simulink library "app"  (R2021b)
settings: Solver=VariableStepAuto  StartTime=0.0  StopTime=10.0  RelTol=1e-3
undefined symbols (not defined in the file): C_TASK_10MS_S, C_TASK_5MS_S, slcm
libraries: acc x1, apm x1, bcm x1, ddm x1, dhp x1, dkc x1, dsc x1, nmm x1, pmm x1, scp x1, sys x1, thc x1
settings Model: Creator=jc19  LastModifiedBy=FVT22115
settings SolverCC: AlgebraicLoopSolver=TrustRegion
settings DataIOCC: SaveFormat=Array  SignalLoggingSaveFormat=ModelDataLogs  ReturnWorkspaceOutputs=off
settings OptimizationCC: BlockReduction=off  BooleanDataType=off
settings DebuggingCC: SaveWithParameterizedLinksMsg=none  UnderspecifiedInitializationDetection=Classic  MergeDetectMultiDrivingBlocksExec=none  SignalResolutionControl=TryResolveAllWithWarning  SFMachineParentedDataDiag=warning
settings HardwareCC: TargetUnknown=on
settings ModelReferenceCC: PropagateSignalLabelsOutOfModel=off
settings SFSimCC: SimUseLocalCustomCode=off
settings RTWCC: RTWUseLocalCustomCode=off
settings ConfigComp: CovMetricSettings=dw  CovSaveCumulativeToWorkspaceVar=on  CovSaveSingleToWorkspaceVar=on

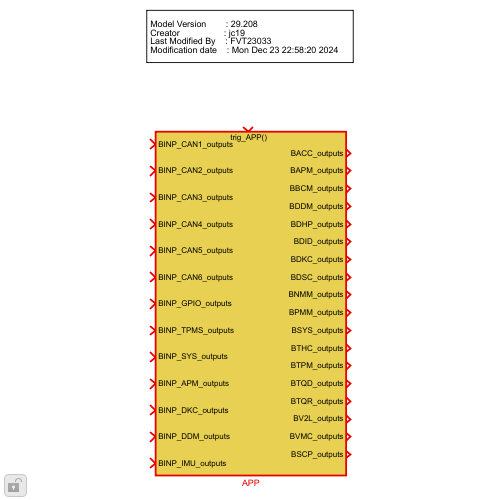
[thumbnail: Simulink's stored preview of the top-level diagram]
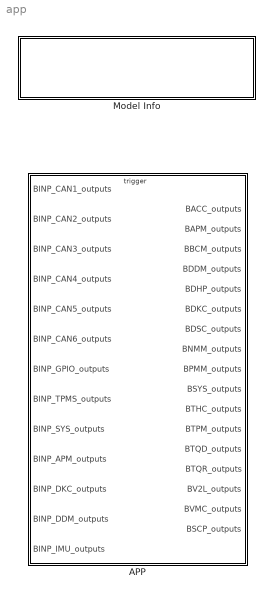
== system app ==
  APP : Subsystem
  Model Info : Subsystem  LoadFcn=slcm LoadBlock;  InitFcn=slcm('UpdateAllCMBlocksInThisModelInit')  mask(CMBlock){InitialSaveTempField=, InitialBlockCM=None, BlockCM=None, Frame=on, SaveTempField=, DisplayStringWithTags=|, MaskDisplayString=Model Version        : 29.221\nCreator                  : jc19\nLast Modified By    : FVT23131\nModification date    : Fri Apr 18 09:47:03 2025, HorizontalTextAlignment=Left, LeftAlignmentValue=0.02, SourceBlockDiagram=app, TagMaxNumber=20, CMTag1=, CMTag2=, CMTag3=, CMTag4=, CMTag5=, CMTag6=, CMTag7=, CMTag8=, CMTag9=, CMTag10=, CMTag11=, CMTag12=, CMTag13=, CMTag14=, CMTag15=, CMTag16=, CMTag17=, CMTag18=, CMTag19=, CMTag20=}
      mask DisplayStringWithTags=|
      | Model Version        : %<ModelVersion>
      | Creator                  : %<Creator>
      | Last Modified By    : %<LastModifiedBy>
      | Modification date    : %<LastModificationDate>
      mask help: This block allows revision control information to be displayed within the model.
      settings: CopyFcn=slcm CopyBlock;  DeleteFcn=slcm Cancel;  PostSaveFcn=slcm('UpdateAllCMBlocksInThisModel')  NameChangeFcn=slcm Rename;  OpenFcn=slcm
      mask Display: text(str2num(LeftAlignmentValue), 0.5, MaskDisplayString, 'HorizontalAlignment', HorizontalTextAlignment)

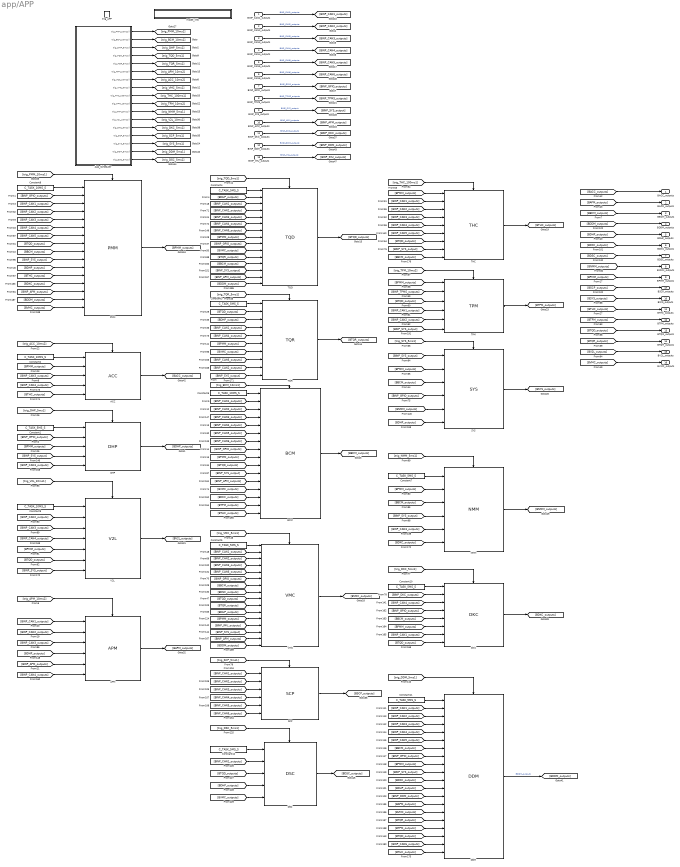
== system app/APP ==
  BINP_CAN1_outputs : Inport  OutDataTypeStr=Bus: BINP_CAN1_outputs
  BINP_CAN2_outputs : Inport  Port=2  OutDataTypeStr=Bus: BINP_CAN2_outputs
  BINP_CAN3_outputs : Inport  Port=3  OutDataTypeStr=Bus: BINP_CAN3_outputs
  BINP_CAN4_outputs : Inport  Port=4  OutDataTypeStr=Bus: BINP_CAN4_outputs
  BINP_CAN5_outputs : Inport  Port=5  OutDataTypeStr=Bus: BINP_CAN5_outputs
  BINP_CAN6_outputs : Inport  Port=6  OutDataTypeStr=Bus: BINP_CAN6_outputs
  BINP_GPIO_outputs : Inport  Port=7  OutDataTypeStr=Bus: BINP_GPIO_outputs
  BINP_TPMS_outputs : Inport  Port=8  OutDataTypeStr=Bus: BINP_TPMS_outputs
  BINP_SYS_outputs : Inport  Port=9  OutDataTypeStr=Bus: BINP_SYS_outputs
  BINP_APM_outputs : Inport  Port=10  OutDataTypeStr=Bus: BINP_APM_outputs
  BINP_DKC_outputs : Inport  Port=11  OutDataTypeStr=Bus: BINP_DKC_outputs
  BINP_DDM_outputs : Inport  Port=12  OutDataTypeStr=Bus: BINP_DDM_outputs
  BINP_IMU_outputs : Inport  Port=13  OutDataTypeStr=Bus: BINP_IMU_outputs
  trig_APP : TriggerPort  TriggerType=function-call  VariantControl=(inherit)
  ACC : acc/ACC  SystemSampleTime=-1  VariantActivationTime=update diagram  Latency=0  AutoFrameSizeCalculation=off
  APM : apm/APM  SystemSampleTime=-1  VariantActivationTime=update diagram  Latency=0  AutoFrameSizeCalculation=off
  App_Scheduler : Stateflow chart  TreatAsAtomicUnit=on
  BCM : bcm/BCM  SystemSampleTime=-1  VariantActivationTime=update diagram  Latency=0  AutoFrameSizeCalculation=off
  Constant{1,3..5,7,10..12} (8 alike) : Constant  Value=C_TASK_5MS_S  OutDataTypeStr=single
  Constant{2,6,8..9} (4 alike) : Constant  Value=C_TASK_10MS_S  OutDataTypeStr=single
  DDM : ddm/DDM  SystemSampleTime=-1  VariantActivationTime=update diagram  Latency=0  AutoFrameSizeCalculation=off
  DHP : dhp/DHP  SystemSampleTime=-1  VariantActivationTime=update diagram  Latency=0  AutoFrameSizeCalculation=off
  DKC : dkc/DKC  SystemSampleTime=-1  VariantActivationTime=update diagram  Latency=0  AutoFrameSizeCalculation=off
  DSC : dsc/DSC  SystemSampleTime=-1  VariantActivationTime=update diagram  Latency=0  AutoFrameSizeCalculation=off
  NMM : nmm/NMM  SystemSampleTime=-1  VariantActivationTime=update diagram  Latency=0  AutoFrameSizeCalculation=off
  PMM : pmm/PMM  SystemSampleTime=-1  VariantActivationTime=update diagram  Latency=0  AutoFrameSizeCalculation=off
  SCP : scp/SCP  SystemSampleTime=-1  VariantActivationTime=update diagram  Latency=0  AutoFrameSizeCalculation=off
  SYS : sys/SYS  SystemSampleTime=-1  VariantActivationTime=update diagram  Latency=0  AutoFrameSizeCalculation=off
  THC : thc/THC  SystemSampleTime=-1  VariantActivationTime=update diagram  Latency=0  AutoFrameSizeCalculation=off
  TPM : tpm/TPM  SystemSampleTime=-1  VariantActivationTime=update diagram  Latency=0  AutoFrameSizeCalculation=off
  TQD : tqd/TQD  SystemSampleTime=-1  VariantActivationTime=update diagram  Latency=0  AutoFrameSizeCalculation=off
  TQR : tqr/TQR  SystemSampleTime=-1  VariantActivationTime=update diagram  Latency=0  AutoFrameSizeCalculation=off
  V2L : v2l/V2L  SystemSampleTime=-1  VariantActivationTime=update diagram  Latency=0  AutoFrameSizeCalculation=off
  VMC : vmc/VMC  SystemSampleTime=-1  VariantActivationTime=update diagram  Latency=0  AutoFrameSizeCalculation=off
  model_info : Subsystem  LoadFcn=slcm LoadBlock;  InitFcn=slcm('UpdateAllCMBlocksInThisModelInit')  mask(CMBlock){InitialSaveTempField=, InitialBlockCM=None, BlockCM=None, Frame=on, SaveTempField=, DisplayStringWithTags=$Id: app.mdl 2023 2013-03-20 03:40:02Z wxia $, MaskDisplayString=$Id: app.mdl 2023 2013-03-20 03:40:02Z wxia $, HorizontalTextAlignment=Center, LeftAlignmentValue=0.5, SourceBlockDiagram=app, TagMaxNumber=20, CMTag1=, CMTag2=, CMTag3=, CMTag4=, CMTag5=, CMTag6=, CMTag7=, CMTag8=, CMTag9=, CMTag10=, CMTag11=, CMTag12=, CMTag13=, CMTag14=, CMTag15=, CMTag16=, CMTag17=, CMTag18=, CMTag19=, CMTag20=}
      mask help: This block allows revision control information to be displayed within the model.
      settings: CopyFcn=slcm CopyBlock;  DeleteFcn=slcm Cancel;  PostSaveFcn=slcm('UpdateAllCMBlocksInThisModel')  NameChangeFcn=slcm Rename;  OpenFcn=slcm
      mask Display: text(str2num(LeftAlignmentValue), 0.5, MaskDisplayString, 'HorizontalAlignment', HorizontalTextAlignment)
  BACC_outputs : Outport  OutDataTypeStr=Bus: BACC_outputs  VectorParamsAs1DForOutWhenUnconnected=off
  BAPM_outputs : Outport  Port=2  OutDataTypeStr=Bus: BAPM_outputs
  BBCM_outputs : Outport  Port=3  OutDataTypeStr=Bus: BBCM_outputs  VectorParamsAs1DForOutWhenUnconnected=off
  BDDM_outputs : Outport  Port=4  OutDataTypeStr=Bus: BDDM_outputs  VectorParamsAs1DForOutWhenUnconnected=off
  BDHP_outputs : Outport  Port=5  OutDataTypeStr=Bus: BDHP_outputs  VectorParamsAs1DForOutWhenUnconnected=off
  BDKC_outputs : Outport  Port=6  OutDataTypeStr=Bus: BDKC_outputs  VectorParamsAs1DForOutWhenUnconnected=off
  BDSC_outputs : Outport  Port=7  OutDataTypeStr=Bus: BDSC_outputs  VectorParamsAs1DForOutWhenUnconnected=off
  BNMM_outputs : Outport  Port=8  OutDataTypeStr=Bus: BNMM_outputs  VectorParamsAs1DForOutWhenUnconnected=off
  BPMM_outputs : Outport  Port=9  OutDataTypeStr=Bus: BPMM_outputs  VectorParamsAs1DForOutWhenUnconnected=off
  BSYS_outputs : Outport  Port=10  OutDataTypeStr=Bus: BSYS_outputs  VectorParamsAs1DForOutWhenUnconnected=off
  BTHC_outputs : Outport  Port=11  OutDataTypeStr=Bus: BTHC_outputs  VectorParamsAs1DForOutWhenUnconnected=off
  BTPM_outputs : Outport  Port=12  OutDataTypeStr=Bus: BTPM_outputs  VectorParamsAs1DForOutWhenUnconnected=off
  BTQD_outputs : Outport  Port=13  OutDataTypeStr=Bus: BTQD_outputs  VectorParamsAs1DForOutWhenUnconnected=off
  BTQR_outputs : Outport  Port=14  OutDataTypeStr=Bus: BTQR_outputs  VectorParamsAs1DForOutWhenUnconnected=off
  BV2L_outputs : Outport  Port=15  OutDataTypeStr=Bus: BV2L_outputs  VectorParamsAs1DForOutWhenUnconnected=off
  BVMC_outputs : Outport  Port=16  OutDataTypeStr=Bus: BVMC_outputs  VectorParamsAs1DForOutWhenUnconnected=off
  BSCP_outputs : Outport  Port=17  OutDataTypeStr=Bus: BSCP_outputs  VectorParamsAs1DForOutWhenUnconnected=off
  wires:
  NMM/1 -> [BNMM_outputs]
  [trig_NMM_5ms1] -> NMM/Trigger
  Constant7/1 -> NMM/1
  DHP/1 -> [BDHP_outputs]
  Constant1/1 -> DHP/1
  [BINP_GPIO_outputs] -> DHP/2
  BINP_CAN1_outputs/1 -> [BINP_CAN1_outputs]  "BINP_CAN1_outputs"
  PMM/1 -> [BPMM_outputs]
  ACC/1 -> [BACC_outputs]
  [trig_PMM_10ms1] -> PMM/Trigger
  TQD/1 -> [BTQD_outputs]
  TQR/1 -> [BTQR_outputs]
  [BTQD_outputs] -> TQR/2
  Constant2/1 -> ACC/1
  [trig_BCM_10ms1] -> BCM/Trigger
  BCM/1 -> [BBCM_outputs]
  BINP_CAN2_outputs/1 -> [BINP_CAN2_outputs]  "BINP_CAN2_outputs"
  BINP_CAN3_outputs/1 -> [BINP_CAN3_outputs]  "BINP_CAN3_outputs"
  BINP_CAN4_outputs/1 -> [BINP_CAN4_outputs]  "BINP_CAN4_outputs"
  BINP_GPIO_outputs/1 -> [BINP_GPIO_outputs]  "BINP_GPIO_outputs"
  [trig_TQD_5ms1] -> TQD/Trigger
  [BPMM_outputs] -> DHP/3
  [trig_DHP_5ms1] -> DHP/Trigger
  BINP_CAN5_outputs/1 -> [BINP_CAN5_outputs]  "BINP_CAN5_outputs"
  [trig_TQR_5ms1] -> TQR/Trigger
  Constant3/1 -> TQR/1
  [BDHP_outputs] -> TQR/3
  [BINP_CAN1_outputs] -> TQR/4
  [trig_ACC_10ms2] -> ACC/Trigger
  [BINP_CAN3_outputs] -> ACC/3
  [BPMM_outputs] -> ACC/2
  [trig_VMC_5ms1] -> VMC/Trigger
  Constant5/1 -> VMC/1
  VMC/1 -> [BVMC_outputs]
  THC/1 -> [BTHC_outputs]
  [BPMM_outputs] -> THC/1
  [trig_THC_100ms1] -> THC/Trigger
  BINP_TPMS_outputs/1 -> [BINP_TPMS_outputs]  "BINP_TPMS_outputs"
  [trig_TPM_10ms2] -> TPM/Trigger
  [BPMM_outputs] -> TPM/1
  [BINP_TPMS_outputs] -> TPM/2
  [BTQD_outputs] -> TPM/3
  [BINP_CAN1_outputs] -> TPM/4
  [BINP_CAN2_outputs] -> TPM/5
  TPM/1 -> [BTPM_outputs]
  SYS/1 -> [BSYS_outputs]
  [BINP_CAN4_outputs] -> TQR/5
  [BPMM_outputs] -> TQR/6
  BINP_SYS_outputs/1 -> [BINP_SYS_output]  "BINP_SYS_output"
  Constant9/1 -> V2L/1
  [BINP_CAN3_outputs] -> V2L/3
  [BINP_CAN2_outputs] -> V2L/2
  [trig_V2L_10ms1] -> V2L/Trigger
  V2L/1 -> [BV2L_outputs]
  APM/1 -> [BAPM_outputs]
  [trig_APM_10ms2] -> APM/Trigger
  [BINP_CAN1_outputs] -> APM/1
  [BINP_CAN2_outputs] -> APM/2
  BINP_APM_outputs/1 -> [BINP_APM_outputs]  "BINP_APM_outputs"
  [trig_SYS_5ms1] -> SYS/Trigger
  [BINP_CAN3_outputs] -> APM/3
  [BVMC_outputs] -> TQR/7
  Constant8/1 -> PMM/1
  [BINP_CAN1_outputs] -> PMM/3
  [BINP_CAN4_outputs] -> PMM/6
  [BINP_GPIO_outputs] -> PMM/2
  [BINP_CAN3_outputs] -> PMM/5
  [BINP_CAN5_outputs] -> PMM/7
  [BTQD_outputs] -> PMM/8
  [BBCM_outputs] -> PMM/9
  [BINP_SYS_output] -> PMM/10
  [BINP_CAN2_outputs] -> PMM/4
  [BDHP_outputs] -> PMM/11
  [BPMM_outputs] -> NMM/2
  [BBCM_outputs] -> NMM/3
  [BINP_SYS_output] -> NMM/4
  [BTHC_outputs] -> PMM/12
  App_Scheduler/3(trig_DHP_5ms1()) -> [trig_DHP_5ms1]
  App_Scheduler/4(trig_TQD_5ms1()) -> [trig_TQD_5ms1]
  App_Scheduler/8(trig_VMC_5ms1()) -> [trig_VMC_5ms1]
  App_Scheduler/15(trig_SYS_5ms1()) -> [trig_SYS_5ms1]
  App_Scheduler/2(trig_BCM_10ms1()) -> [trig_BCM_10ms1]
  App_Scheduler/12(trig_V2L_10ms1()) -> [trig_V2L_10ms1]
  App_Scheduler/5(trig_TQR_5ms1()) -> [trig_TQR_5ms1]
  App_Scheduler/9(trig_THC_100ms1()) -> [trig_THC_100ms1]
  App_Scheduler/6(trig_APM_10ms2()) -> [trig_APM_10ms2]
  App_Scheduler/7(trig_ACC_10ms2()) -> [trig_ACC_10ms2]
  App_Scheduler/11(trig_NMM_5ms1()) -> [trig_NMM_5ms1]
  App_Scheduler/10(trig_TPM_10ms2()) -> [trig_TPM_10ms2]
  App_Scheduler/1(trig_PMM_10ms1()) -> [trig_PMM_10ms1]
  App_Scheduler/13(trig_DKC_5ms1()) -> [trig_DKC_5ms1]
  App_Scheduler/14(trig_SCP_5ms1()) -> [trig_SCP_5ms1]
  BINP_DKC_outputs/1 -> [BINP_DKC_outputs]  "BINP_DKC_outputs"
  [trig_DKC_5ms1] -> DKC/Trigger
  Constant10/1 -> DKC/1
  [BINP_DKC_outputs] -> DKC/2
  [BINP_CAN3_outputs] -> SCP/3
  [BINP_CAN2_outputs] -> SCP/2
  [BINP_CAN1_outputs] -> SCP/1
  [BINP_CAN4_outputs] -> SCP/4
  [BINP_CAN5_outputs] -> SCP/5
  [trig_SCP_5ms1] -> SCP/Trigger
  SCP/1 -> [BSCP_outputs]
  DKC/1 -> [BDKC_outputs]
  [BSYS_outputs] -> BSYS_outputs/1
  [BTQR_outputs] -> BTQR_outputs/1
  [BAPM_outputs] -> BAPM_outputs/1
  [BPMM_outputs] -> BPMM_outputs/1
  [BV2L_outputs] -> BV2L_outputs/1
  [BTQD_outputs] -> BTQD_outputs/1
  [BDHP_outputs] -> BDHP_outputs/1
  [BTPM_outputs] -> BTPM_outputs/1
  [BDKC_outputs] -> BDKC_outputs/1
  [BACC_outputs] -> BACC_outputs/1
  [BNMM_outputs] -> BNMM_outputs/1
  [BVMC_outputs] -> BVMC_outputs/1
  [BSCP_outputs] -> BSCP_outputs/1
  [BBCM_outputs] -> BBCM_outputs/1
  [BTHC_outputs] -> BTHC_outputs/1
  [BINP_SYS_output] -> SYS/1
  [BPMM_outputs] -> SYS/2
  [BBCM_outputs] -> SYS/3
  [BINP_GPIO_outputs] -> SYS/4
  App_Scheduler/16(trig_DDM_5ms1()) -> [trig_DDM_5ms1]
  [trig_DDM_5ms1] -> DDM/Trigger
  [BDDM_outputs] -> BDDM_outputs/1
  BINP_DDM_outputs/1 -> [BINP_DDM_outputs]  "BINP_DDM_outputs"
  [BINP_CAN1_outputs] -> VMC/2
  [BINP_CAN2_outputs] -> VMC/3
  [BINP_CAN3_outputs] -> VMC/4
  App_Scheduler/17(trig_DSC_5ms1()) -> [trig_DSC_5ms1]
  [trig_DSC_5ms1] -> DSC/Trigger
  Constant12/1 -> DSC/1
  [BINP_CAN1_outputs] -> DSC/2
  [BTQD_outputs] -> DSC/3
  [BDHP_outputs] -> DSC/4
  [BVMC_outputs] -> DSC/5
  DSC/1 -> [BDSC_outputs]
  BINP_CAN6_outputs/1 -> [BINP_CAN6_outputs]  "BINP_CAN6_outputs"
  [BDSC_outputs] -> BDSC_outputs/1
  Constant6/1 -> BCM/1
  [BINP_CAN1_outputs] -> BCM/2
  [BINP_CAN2_outputs] -> BCM/3
  Constant11/1 -> DDM/1
  [BINP_CAN1_outputs] -> DDM/2
  [BINP_CAN2_outputs] -> DDM/3
  [BINP_CAN3_outputs] -> DDM/4
  [BINP_CAN4_outputs] -> DDM/5
  [BINP_CAN5_outputs] -> DDM/6
  [BBCM_outputs] -> DDM/7
  [BINP_GPIO_outputs] -> DDM/8
  [BPMM_outputs] -> DDM/9
  [BINP_SYS_output] -> DDM/10
  [BDKC_outputs] -> DDM/11
  [BDHP_outputs] -> DDM/12
  [BINP_DDM_outputs] -> DDM/13
  [BAPM_outputs] -> DDM/14
  [BVMC_outputs] -> DDM/15
  [BTQR_outputs] -> DDM/16
  [BTPM_outputs] -> DDM/17
  [BINP_CAN3_outputs] -> NMM/5
  [BINP_CAN1_outputs] -> THC/2
  [BINP_CAN2_outputs] -> THC/3
  [BINP_CAN3_outputs] -> THC/4
  [BINP_CAN4_outputs] -> THC/5
  [BINP_SYS_output] -> THC/8
  [BTQD_outputs] -> THC/7
  [BINP_CAN5_outputs] -> THC/6
  [BINP_CAN4_outputs] -> DKC/3
  DDM/1 -> [BDDM_outputs]  "BDDM_outputs"
  BINP_IMU_outputs/1 -> [BINP_IMU_outputs]  "BINP_IMU_outputs"
  [BTQD_outputs] -> DDM/18
  [BNMM_outputs] -> SYS/5
  [BINP_CAN6_outputs] -> SCP/6
  [BINP_SYS_output] -> DHP/4
  Constant4/1 -> TQD/1
  [BDHP_outputs] -> TQD/2
  [BINP_CAN1_outputs] -> TQD/3
  [BINP_CAN2_outputs] -> TQD/4
  [BINP_CAN3_outputs] -> TQD/5
  [BINP_CAN4_outputs] -> TQD/6
  [BINP_CAN3_outputs] -> BCM/4
  [BINP_CAN4_outputs] -> BCM/5
  [BINP_CAN5_outputs] -> BCM/6
  [BINP_CAN6_outputs] -> BCM/7
  [BINP_GPIO_outputs] -> BCM/8
  [BPMM_outputs] -> BCM/9
  [BTQD_outputs] -> BCM/10
  [BINP_SYS_output] -> BCM/11
  [BINP_APM_outputs] -> BCM/12
  [BINP_APM_outputs] -> APM/5
  [BDHP_outputs] -> APM/4
  [BINP_CAN6_outputs] -> TQD/7
  [BPMM_outputs] -> TQD/8
  [BTQR_outputs] -> TQD/11
  [BINP_GPIO_outputs] -> TQD/9
  [BVMC_outputs] -> TQD/10
  [BBCM_outputs] -> TQD/12
  [BINP_SYS_output] -> TQD/13
  [BINP_CAN6_outputs] -> VMC/5
  [BINP_GPIO_outputs] -> VMC/6
  [BBCM_outputs] -> VMC/7
  [BDSC_outputs] -> VMC/8
  [BTQD_outputs] -> VMC/9
  [BTQR_outputs] -> VMC/10
  [BDHP_outputs] -> VMC/11
  [BPMM_outputs] -> VMC/12
  [BINP_IMU_outputs] -> VMC/13
  [BINP_SYS_output] -> VMC/14
  [BVMC_outputs] -> BCM/13
  [BDKC_outputs] -> BCM/14
  [BDKC_outputs] -> PMM/13
  [BTPM_outputs] -> BCM/15
  [BTHC_outputs] -> BCM/16
  [BINP_CAN6_outputs] -> TQR/8
  [BINP_APM_outputs] -> TQD/14
  [BINP_CAN3_outputs] -> DHP/5
  [BINP_CAN4_outputs] -> APM/6
  [BINP_APM_outputs] -> PMM/14
  [BINP_GPIO_outputs] -> DKC/4
  [BBCM_outputs] -> DKC/5
  [BPMM_outputs] -> DKC/6
  [BINP_CAN1_outputs] -> DKC/7
  [BTQD_outputs] -> DKC/8
  [BINP_APM_outputs] -> VMC/15
  [BINP_CAN2_outputs] -> TQR/9
  [BTQD_outputs] -> V2L/6
  [BPMM_outputs] -> V2L/5
  [BINP_CAN4_outputs] -> V2L/4
  [BINP_SYS_output] -> V2L/7
  [BDHP_outputs] -> SYS/6
  [BINP_SYS_output] -> TQR/10
  [BDKC_outputs] -> NMM/6
  [BDDM_outputs] -> TQD/15
  [BDDM_outputs] -> PMM/15
  [BVMC_outputs] -> PMM/16
  [BINP_CAN6_outputs] -> DDM/19
  [BDDM_outputs] -> VMC/16
  [BINP_SYS_output] -> TPM/6
  [BINP_CAN4_outputs] -> ACC/4
  [BTHC_outputs] -> ACC/5
  [BTHC_outputs] -> DDM/20
  [BBCM_outputs] -> THC/9

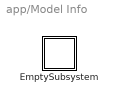
== system app/Model Info ==
  EmptySubsystem : Subsystem

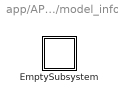
== system app/APP/model_info ==
  EmptySubsystem : Subsystem

== system app/Model Info/EmptySubsystem ==

== system app/APP/model_info/EmptySubsystem ==

== stateflow chart app/APP/App_Scheduler ==
  state Task_5_10_100ms
    (default) -> (junction 6) : {
        | counter = 0;
        | }
    Task_5_10_100ms -> (junction 6) : {
        | counter++;
        | }
    (junction 6) -> (junction 38) [order 1] : [counter%%2 == 0]  /* 10ms trigger #1*/
    (junction 6) -> (junction 44) [order 2]
    (junction 38) -> (junction 40) : {
        | trig_PMM_10ms1;
        | trig_BCM_10ms1;
        | trig_V2L_10ms1;
        | }
    (junction 40) -> (junction 44)
    (junction 44) -> (junction 63)
    (junction 63) -> (junction 107) [order 1] : %[VPMM_PowerSta_enum == ENUM_POWERSTA_ON ||...
        | %VPMM_PowerSta_enum == ENUM_POWERSTA_READY]
    (junction 63) -> (junction 69) [order 2]
    (junction 107) -> (junction 108) : {
        | trig_DHP_5ms1;
        | trig_TQD_5ms1;
        | trig_TQR_5ms1;
        | trig_VMC_5ms1;
        | trig_NMM_5ms1;
        | trig_SCP_5ms1;
        | trig_DKC_5ms1;
        | trig_DSC_5ms1;
        | trig_DDM_5ms1;
        | }
    (junction 108) -> (junction 69)
    (junction 69) -> (junction 115)
    (junction 115) -> (junction 113) [order 1] : [counter%%2 == 1]  /* 10ms trigger #2*/
    (junction 115) -> (junction 124) [order 2]
    (junction 113) -> (junction 117) : {
        | trig_APM_10ms2;
        | trig_ACC_10ms2;
        | trig_TPM_10ms2;
        | }
    (junction 117) -> (junction 124)
    (junction 124) -> (junction 131)
    (junction 131) -> (junction 133) [order 1] : [counter%% 20 == 0]  /*100ms trigger #1*/
    (junction 131) -> (junction 137) [order 2]
    (junction 133) -> (junction 135) : {
        |  trig_THC_100ms1;
        |  counter = 0;
        |  }
    (junction 135) -> (junction 137)
    (junction 137) -> (junction 154) : {
        |  trig_SYS_5ms1;
        | }
  data: counter local double
  events: trig_PMM_10ms1 output FUNCTION_CALL_EVENT; trig_BCM_10ms1 output FUNCTION_CALL_EVENT; trig_DHP_5ms1 output FUNCTION_CALL_EVENT; trig_TQD_5ms1 output FUNCTION_CALL_EVENT; trig_TQR_5ms1 output FUNCTION_CALL_EVENT; trig_APM_10ms2 output FUNCTION_CALL_EVENT; trig_ACC_10ms2 output FUNCTION_CALL_EVENT; trig_VMC_5ms1 output FUNCTION_CALL_EVENT; trig_THC_100ms1 output FUNCTION_CALL_EVENT; trig_TPM_10ms2 output FUNCTION_CALL_EVENT; trig_NMM_5ms1 output FUNCTION_CALL_EVENT; trig_V2L_10ms1 output FUNCTION_CALL_EVENT; trig_DKC_5ms1 output FUNCTION_CALL_EVENT; trig_SCP_5ms1 output FUNCTION_CALL_EVENT; trig_SYS_5ms1 output FUNCTION_CALL_EVENT; trig_DDM_5ms1 output FUNCTION_CALL_EVENT; trig_DSC_5ms1 output FUNCTION_CALL_EVENT
